simulink model "W3P2"  (R2020b)
settings: Solver=VariableStepAuto  StartTime=0.0  StopTime=10.0  RelTol=1e-3
settings Model: Creator=saadh  LastModifiedBy=saadh

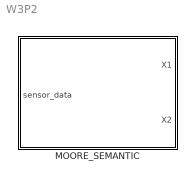
== system W3P2 ==
  MOORE_SEMANTIC : Stateflow chart  TreatAsAtomicUnit=on

== stateflow chart W3P2/MOORE_SEMANTIC ==
  state STOP_to_GO
    X1 = RED;
    X2 = YELLOW;
  state STOP
    X1 = RED;
    X2 = GREEN;
  state STOP_for_Traffic
    X1 = RED;
    X2 = GREEN;
  state GO
    X1 = GREEN;
    X2 = RED;
  state GO_to_STOP
    X1 = YELLOW;
    X2 = RED;
  (default) -> STOP
  STOP_for_Traffic -> STOP_to_GO : [sensor_data]
  STOP -> STOP_for_Traffic : after(20,tick)
  STOP_to_GO -> GO : after(3,tick)
  GO_to_STOP -> STOP : after(3,tick)
  GO -> GO_to_STOP : after(10,tick)
  data: sensor_data input; X1 output; X2 output; GREEN constant double =3; RED constant double =1; YELLOW constant double =2
